simulink model "HW02_2"  (R2021a)
settings: Solver=FixedStepAuto  StartTime=0.0  StopTime=inf  FixedStep=0.001  RelTol=1e-3  EnableMultiTasking=on
libraries: raspberrypiBasiclib x2
settings Model: Creator=HP  LastModifiedBy=ku347
settings SolverCC: PositivePriorityOrder=on
settings OptimizationCC: EnhancedBackFolding=on  PassReuseOutputArgsAs=Individual arguments  ZeroExternalMemoryAtStartup=off  ZeroInternalMemoryAtStartup=off  MaxStackSize=64  OptimizeBlockOrder=speed  DifferentSizesBufferReuse=on  OptimizationCustomize=off  EfficientTunableParamExpr=on
settings DebuggingCC: ParameterTunabilityLossMsg=error  UnconnectedInputMsg=none  UnconnectedOutputMsg=none  UnconnectedLineMsg=none
settings HardwareCC: ProdBitPerPointer=32  ProdBitPerSizeT=32  ProdBitPerPtrDiffT=32  ProdLargestAtomicInteger=Long  ProdLargestAtomicFloat=Double  ProdWordSize=32  ProdLongLongMode=on  ProdHWDeviceType=ARM Compatible->ARM Cortex  UseEmbeddedCoderFeatures=off
settings RTWCC: SystemTargetFile=ert.tlc  HardwareBoard=Raspberry Pi  TLCOptions="-aInlineSetEventsForThisBaseRateFcn=TLC_FALSE -aSuppressMultiTaskScheduler=TLC_FALSE  -aRateBasedStepFcn=0"  TemplateMakefile=ert_default_tmf  Toolchain=GNU GCC Embedded Linux  BuildConfiguration=Specify  DLArmComputeVersion=20.02.1
settings CodeAppCC: ForceParamTrailComments=on  IgnoreCustomStorageClasses=off  OperatorAnnotations=on  SimulinkDataObjDesc=on  SFDataObjDesc=on  InsertBlockDesc=on
settings ERTTargetCC: SupportNonInlinedSFcns=on  SupportVariableSizeSignals=on  ExtModeTransport=2  ExtModeStaticAlloc=on  ExtModeMexFile=ext_xcp  ExtModeIntrfLevel=Level2 - Open

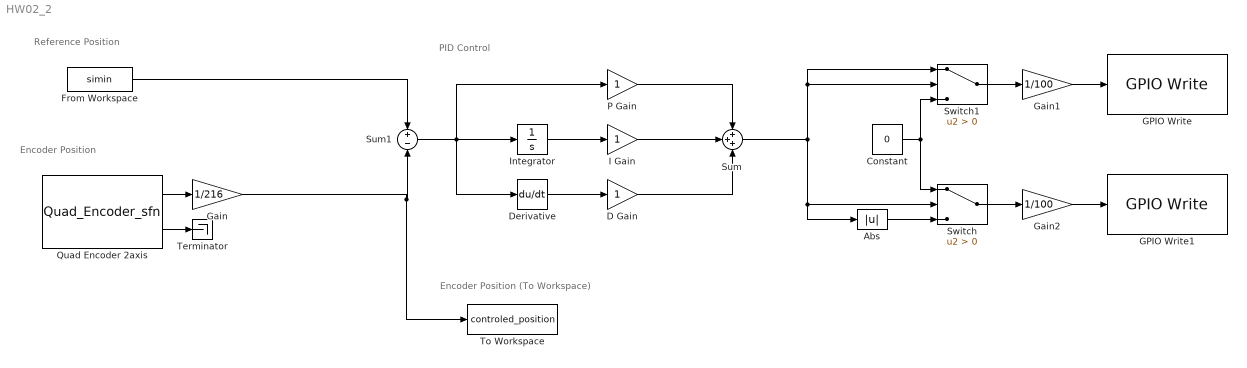
== system HW02_2 ==
  note: Encoder Position (To Workspace)
  note: Encoder Position
  note: Reference Position
  note: PID Control
  Abs : Abs
  Constant : Constant  Value=0
  D Gain : Gain
  Derivative : Derivative
  From Workspace : FromWorkspace  VariableName=simin  SampleTime=-1
  GPIO Write : raspberrypiBasiclib/GPIO Write  board=Pi 4 Model B  gpio=5  direction=Output  blockPlatform=Raspberry Pi
      settings: SourceProductBaseCode=RASPPI
  GPIO Write1 : raspberrypiBasiclib/GPIO Write  board=Pi 4 Model B  gpio=6  direction=Output  blockPlatform=Raspberry Pi
      settings: SourceProductBaseCode=RASPPI
  Gain : Gain  Gain=1/216
  Gain1 : Gain  Gain=1/100
  Gain2 : Gain  Gain=1/100
  I Gain : Gain
  Integrator : Integrator
  P Gain : Gain
  Quad Encoder 2axis : S-Function  InitFcn=try, set_param(gcb,'FunctionName','Quad_Encoder_sfn'), end  FunctionName=Quad_Encoder_sfn  Parameters=uint8(0),uint8(5),uint8(6),uint8(1),uint8(23),uint8(24)  SFunctionModules=Quad_Encoder_sfn_wrapper  SFunctionDeploymentMode=off  EnableBusSupport=off  mask(S-Function Builder){}
      mask init:
      | val = [[.9  0.75 0.75 1 1 .9 .9 1]',[1 1 0.75 0.75 .9 .9 1 .9]'];try , sys = get_param(gcb,'SfunBuilderFcnName');if isempty(sys), sys = get_param(gcb,'FunctionName'); end,catch, sys = get_param(gcb,'FunctionName'); end
      settings: CopyFcn=set_param(gcbh,'LinkStatus','none')  PreSaveFcn=try, set_param(gcb,'FunctionName','Quad_Encoder_sfn'), end  OpenFcn=sfunctionwizard(gcbh)
      mask Display:
      | plot(val(:,1),val(:,2))
      | disp(sys)
      | port_label('output',1,'enc_pos1')
      | port_label('output',2,'enc_pos2')
  Sum : Sum  Inputs=+++
  Sum1 : Sum  Inputs=+-
  Switch : Switch  Criteria=u2 > Threshold
  Switch1 : Switch  Criteria=u2 > Threshold
  Terminator : Terminator
  To Workspace : ToWorkspace  VariableName=controled_position  SaveFormat=Structure With Time  SampleTime=0.001
  wires:
  Integrator/1 -> I Gain/1
  Derivative/1 -> D Gain/1
  I Gain/1 -> Sum/2
  P Gain/1 -> Sum/1
  D Gain/1 -> Sum/3
  Quad Encoder 2axis/1 -> Gain/1
  From Workspace/1 -> Sum1/1
  Sum1/1 -> Derivative/1, P Gain/1, Integrator/1
  Quad Encoder 2axis/2 -> Terminator/1
  Constant/1 -> Switch/1, Switch1/3
  Sum/1 -> Abs/1, Switch/2, Switch1/1, Switch1/2
  Abs/1 -> Switch/3
  Switch1/1 -> Gain1/1
  Switch/1 -> Gain2/1
  Gain1/1 -> GPIO Write/1
  Gain2/1 -> GPIO Write1/1
  Gain/1 -> To Workspace/1, Sum1/2
